simulink library "drr"  (Simulink 8.1)
settings: Solver=ode1  StartTime=0.0  StopTime=Inf  FixedStep=0.001  RelTol=1e-3
PostLoadFcn:
  | , if any(exist('dsrtsu_mdlpostloadfcn', 'file') == [2, 3, 6]), try dsrtsu_mdlpostloadfcn('Execute', bdroot); catch fprintf('Error in PostLoadFcn (dsrtsu_mdlpostloadfcn) for model "%s":\n %s\n', bdroot, lasterr); end, end,
undefined symbols (not defined in the file or in its folder): C_TICK_TIME_S, FALSE, KACC_ACCDecelIncLongTimer_s, KACC_ACCDecelIncMedTimer_s, KACC_ACCDecelIncShortTimer_s, KACC_ACCDecelIncSteps_num, KACC_ACCMCHardBrakingThrs_mps2, KACC_ACCMinSetTimeGap_s, KACC_BTSDecelRampDownRollAvgInt_s, KACC_DecelRampDownRollAvgInt_s, KACC_TargetDecelMargin_mps2, KACC_TimeGapIntrusionPerc_perc, TRUE, ZERO_FLOAT, ZERO_INT
libraries: hcu_lib x1, ltd x1
settings Model: DSRTSU_INTERNAL_RTI_VER=450  DSRTSU_INTERNAL_RTI_TYPE=rti1401  RTICANMMDATA=struct('GeneralSetupData',struct('modelroot','D:\ELN150201_TAIWAN\trunk\AdasDragon\software\sw_development\arch\app\acc','generalsettings',struct('filesettings',struct('destfolder',struct('Name','RTICANMM_FILES','Check',1),'buildfolder',struct('Name','.','Check',1),'AbsDestfolder',struct('Name','D:\ELN150201_TAIWAN\trunk\AdasDragon\software\sw_development\arch\app\acc\RTICANMM_FILES'),'AbsBuildfolder',struct('Name','D:\ELN150201_TAIWAN\trunk\AdasDragon\software\sw_development\arch\app\acc'))),'options',struct('addpaths',1,'rmpaths',1,'addtrcexclusion',logical(1),'cannavigator',struct('checkmonitoring',0),'show_usrtrc',0,'use_usrtrc',0),'advanced',struct('options',[1 1 1 1 1 1 1 1 1 1 1 1 1 1 1 1 1 1 1 1 1 1 1 1 1 1 1 1 1 1 1 1 1 1 1 1 1 1 1 1 1 1 1 1 1 1 1 1 1 1 1 1 1 1 1 1 1 1 1 1 1 1 1 1 1 1 1 1 1 1 1 1 1 1 1 1 1 1 1 1 1 1 1 1 1 1 1 1 1 1 1 1 1 1 1 1 1 1 1 1]),'MPSetup',{{}},'modelname','drr','block','drr'))  DSRTSU_INTERNAL_RTIFPGA=40  Creator=AT015411  LastModifiedBy=AT015555

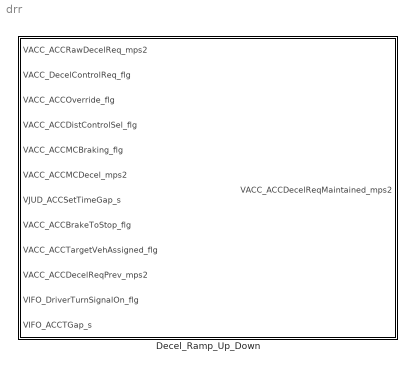
== system drr ==
  Decel_Ramp_Up_Down : Subsystem

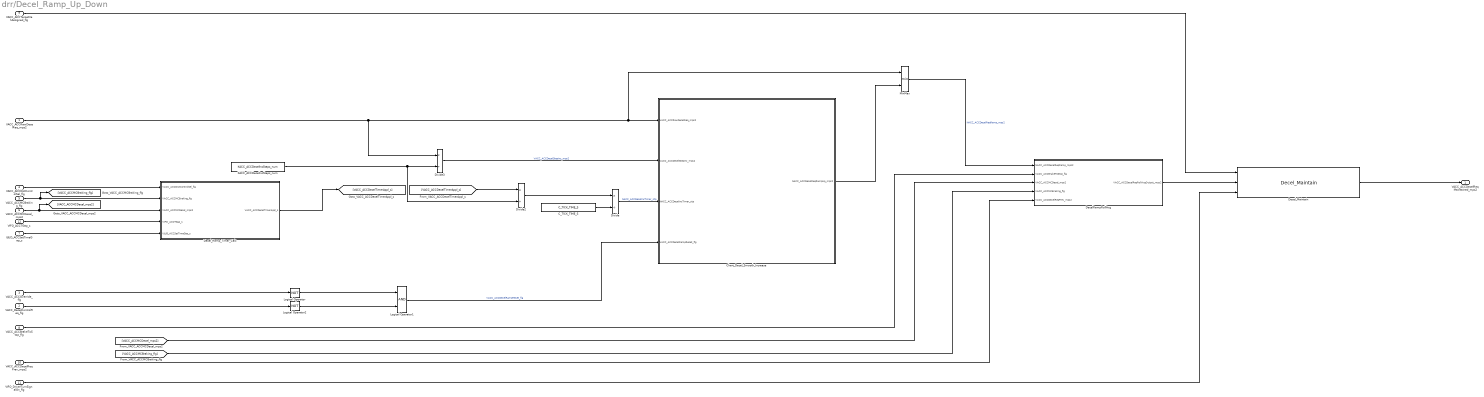
== system drr/Decel_Ramp_Up_Down ==
  VACC_ACCRawDecelReq_mps2 : Inport
  VACC_DecelControlReq_flg : Inport  Port=2
  VACC_ACCOverride_flg : Inport  Port=3
  VACC_ACCDistControlSel_flg : Inport  Port=4
  VACC_ACCMCBraking_flg : Inport  Port=5
  VACC_ACCMCDecel_mps2 : Inport  Port=6
  VJUD_ACCSetTimeGap_s : Inport  Port=7
  VACC_ACCBrakeToStop_flg : Inport  Port=8
  VACC_ACCTargetVehAssigned_flg : Inport  Port=9
  VACC_ACCDecelReqPrev_mps2 : Inport  Port=10
  VIFO_DriverTurnSignalOn_flg : Inport  Port=11
  VIFO_ACCTGap_s : Inport  Port=12
  C_TICK_TIME_S : Constant  Value=C_TICK_TIME_S
  Chart_Decel_Smooth_Increase : Stateflow chart  TreatAsAtomicUnit=on
  DecelRampRollAvg : Subsystem
  Decel_Maintain : ltd/Decel_Maintain
  Decel_Ramp_Timer_Calc : Subsystem
  Divide : Product  Inputs=*/
  Divide2 : Product  Inputs=*/
  Divide3 : Product  Inputs=*/
  KACC_ACCDecelIncSteps_num : Constant  Value=KACC_ACCDecelIncSteps_num
  Logical Operator : Logic  Operator=NOT  AllPortsSameDT=off  OutDataTypeStr=boolean
  Logical Operator1 : Logic  AllPortsSameDT=off  OutDataTypeStr=boolean
  Logical Operator2 : Logic  Operator=NOT  AllPortsSameDT=off  OutDataTypeStr=boolean
  MinMax : MinMax  Inputs=2
  VACC_ACCDecelReqMaintained_mps2 : Outport
  wires:
  Logical Operator2/1 -> Logical Operator1/2
  Chart_Decel_Smooth_Increase/1(NACC_ACCDecelReqRampUp_mps2) -> MinMax/2
  Divide3/1 -> Chart_Decel_Smooth_Increase/2(VACC_ACCDecelStepInc_mps2)  "VACC_ACCDecelStepInc_mps2"
  KACC_ACCDecelIncSteps_num/1 -> Divide2/2, Divide3/2
  Divide/1 -> Chart_Decel_Smooth_Increase/3(NACC_ACCDecelIncTimer_stp)  "NACC_ACCDecelIncTimer_stp"
  C_TICK_TIME_S/1 -> Divide/2
  Divide2/1 -> Divide/1
  VACC_ACCRawDecelReq_mps2/1 -> Divide3/1, MinMax/1, Chart_Decel_Smooth_Increase/1(VACC_ACCRawDecelReq_mps2)
  Logical Operator1/1 -> Chart_Decel_Smooth_Increase/4(VACC_ACCDecelRampReset_flg)  "VACC_ACCDecelRampReset_flg"
  VACC_ACCOverride_flg/1 -> Logical Operator/1
  Logical Operator/1 -> Logical Operator1/1
  VACC_DecelControlReq_flg/1 -> Logical Operator2/1
  [VACC_ACCDecelTimerAppl_s] -> Divide2/1
  VACC_ACCDistControlSel_flg/1 -> Decel_Ramp_Timer_Calc/1(VACC_ACCDistControlSel_flg)
  VIFO_ACCTGap_s/1 -> Decel_Ramp_Timer_Calc/4(VIFO_ACCTGap_s)
  VACC_ACCMCDecel_mps2/1 -> [VACC_ACCMCDecel_mps2], Decel_Ramp_Timer_Calc/3(VACC_ACCMCDecel_mps2)
  VJUD_ACCSetTimeGap_s/1 -> Decel_Ramp_Timer_Calc/5(VJUD_ACCSetTimeGap_s)
  VACC_ACCMCBraking_flg/1 -> [VACC_ACCMCBraking_flg], Decel_Ramp_Timer_Calc/2(VACC_ACCMCBraking_flg)
  Decel_Ramp_Timer_Calc/1(VACC_ACCDecelTimerAppl_s) -> [VACC_ACCDecelTimerAppl_s]
  VACC_ACCBrakeToStop_flg/1 -> DecelRampRollAvg/2(VACC_ACCBrakeToStop_flg)
  MinMax/1 -> DecelRampRollAvg/1(NACC_ACCDecelReqRamp_mps2)  "NACC_ACCDecelReqRamp_mps2"
  VACC_ACCTargetVehAssigned_flg/1 -> Decel_Maintain/1
  [VACC_ACCMCDecel_mps2] -> DecelRampRollAvg/3(VACC_ACCMCDecel_mps2)
  VACC_ACCDecelReqPrev_mps2/1 -> DecelRampRollAvg/5(VACC_ACCDecelReqPrev_mps2)
  DecelRampRollAvg/1(VACC_ACCDecelReqRollAvgOutput_mps2) -> Decel_Maintain/2
  Decel_Maintain/1 -> VACC_ACCDecelReqMaintained_mps2/1
  VIFO_DriverTurnSignalOn_flg/1 -> Decel_Maintain/3
  [VACC_ACCMCBraking_flg] -> DecelRampRollAvg/4(VACC_ACCMCBraking_flg)

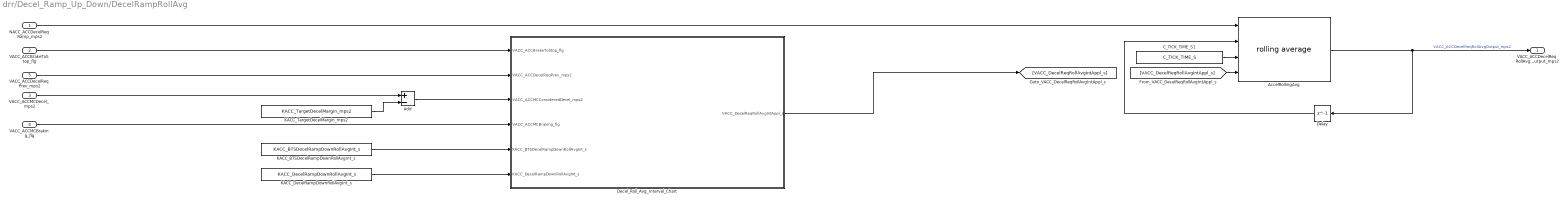
== system drr/Decel_Ramp_Up_Down/DecelRampRollAvg ==
  NACC_ACCDecelReqRamp_mps2 : Inport
  VACC_ACCBrakeToStop_flg : Inport  Port=2
  VACC_ACCMCDecel_mps2 : Inport  Port=3
  VACC_ACCMCBraking_flg : Inport  Port=4
  VACC_ACCDecelReqPrev_mps2 : Inport  Port=5
  AccelRollingAvg : hcu_lib/rolling average
  Add : Sum  Inputs=+-
  C_TICK_TIME_S1 : Constant  Value=C_TICK_TIME_S
  Decel_Roll_Avg_Interval_Chart : Stateflow chart  TreatAsAtomicUnit=on
  Delay : Delay  DelayLength=1
  KACC_BTSDecelRampDownRollAvgInt_s : Constant  Value=KACC_BTSDecelRampDownRollAvgInt_s
  KACC_DecelRampDownRollAvgInt_s : Constant  Value=KACC_DecelRampDownRollAvgInt_s
  KACC_TargetDecelMargin_mps2 : Constant  Value=KACC_TargetDecelMargin_mps2  OutDataTypeStr=single
  VACC_ACCDecelReqRollAvgOutput_mps2 : Outport
  wires:
  Delay/1 -> AccelRollingAvg/2
  KACC_DecelRampDownRollAvgInt_s/1 -> Decel_Roll_Avg_Interval_Chart/6(KACC_DecelRampDownRollAvgInt_s)
  C_TICK_TIME_S1/1 -> AccelRollingAvg/3
  NACC_ACCDecelReqRamp_mps2/1 -> AccelRollingAvg/1
  AccelRollingAvg/1 -> VACC_ACCDecelReqRollAvgOutput_mps2/1, Delay/1  "VACC_ACCDecelReqRollAvgOutput_mps2"
  VACC_ACCBrakeToStop_flg/1 -> Decel_Roll_Avg_Interval_Chart/1(VACC_ACCBrakeToStop_flg)
  KACC_BTSDecelRampDownRollAvgInt_s/1 -> Decel_Roll_Avg_Interval_Chart/5(KACC_BTSDecelRampDownRollAvgInt_s)
  [VACC_DecelReqRollAvgIntAppl_s] -> AccelRollingAvg/4
  VACC_ACCMCDecel_mps2/1 -> Add/1
  VACC_ACCDecelReqPrev_mps2/1 -> Decel_Roll_Avg_Interval_Chart/2(VACC_ACCDecelReqPrev_mps2)
  Decel_Roll_Avg_Interval_Chart/1(VACC_DecelReqRollAvgIntAppl_s) -> [VACC_DecelReqRollAvgIntAppl_s]
  KACC_TargetDecelMargin_mps2/1 -> Add/2
  Add/1 -> Decel_Roll_Avg_Interval_Chart/3(VACC_ACCMCConsideredDecel_mps2)
  VACC_ACCMCBraking_flg/1 -> Decel_Roll_Avg_Interval_Chart/4(VACC_ACCMCBraking_flg)

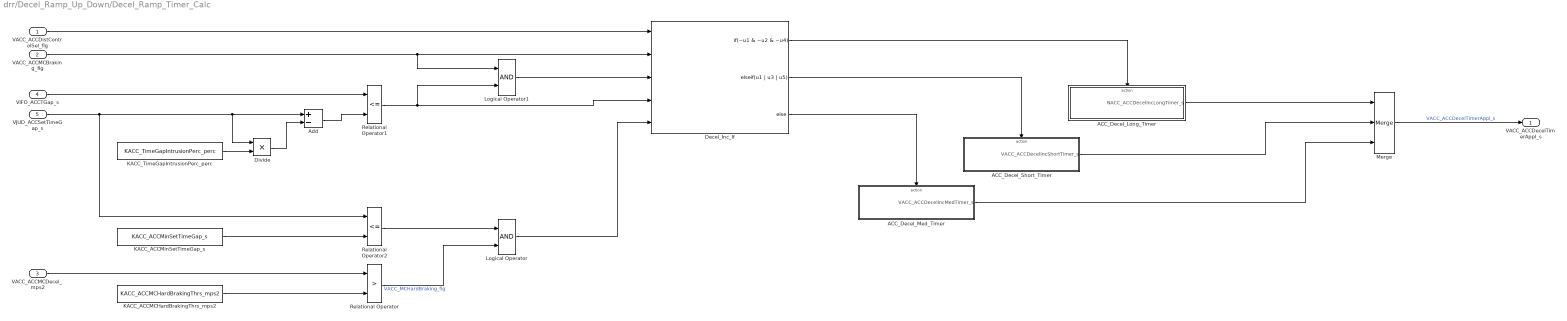
== system drr/Decel_Ramp_Up_Down/Decel_Ramp_Timer_Calc ==
  VACC_ACCDistControlSel_flg : Inport
  VACC_ACCMCBraking_flg : Inport  Port=2
  VACC_ACCMCDecel_mps2 : Inport  Port=3
  VIFO_ACCTGap_s : Inport  Port=4
  VJUD_ACCSetTimeGap_s : Inport  Port=5
  ACC_Decel_Long_Timer : Subsystem  TreatAsAtomicUnit=on
  ACC_Decel_Med_Timer : Subsystem  TreatAsAtomicUnit=on
  ACC_Decel_Short_Timer : Subsystem  TreatAsAtomicUnit=on
  Add : Sum  Inputs=+-
  Decel_Inc_If : If  NumInputs=5  IfExpression=~u1 & ~u2 & ~u4  ElseIfExpressions=u1 | u3 | u5
  Divide : Product  Inputs=**
  KACC_ACCMCHardBrakingThrs_mps2 : Constant  Value=KACC_ACCMCHardBrakingThrs_mps2
  KACC_ACCMinSetTimeGap_s : Constant  Value=KACC_ACCMinSetTimeGap_s
  KACC_TimeGapIntrusionPerc_perc : Constant  Value=KACC_TimeGapIntrusionPerc_perc
  Logical Operator : Logic  AllPortsSameDT=off  OutDataTypeStr=boolean
  Logical Operator1 : Logic  AllPortsSameDT=off  OutDataTypeStr=boolean
  Merge : Merge  Inputs=3
  Relational Operator : RelationalOperator  Operator=>  OutDataTypeStr=boolean
  Relational Operator1 : RelationalOperator  Operator=<=  OutDataTypeStr=boolean
  Relational Operator2 : RelationalOperator  Operator=<=  OutDataTypeStr=boolean
  VACC_ACCDecelTimerAppl_s : Outport
  wires:
  VACC_ACCMCDecel_mps2/1 -> Relational Operator/1
  KACC_ACCMCHardBrakingThrs_mps2/1 -> Relational Operator/2
  VIFO_ACCTGap_s/1 -> Relational Operator1/1
  VJUD_ACCSetTimeGap_s/1 -> Add/1, Divide/1, Relational Operator2/1
  KACC_ACCMinSetTimeGap_s/1 -> Relational Operator2/2
  VACC_ACCDistControlSel_flg/1 -> Decel_Inc_If/1
  VACC_ACCMCBraking_flg/1 -> Logical Operator1/1, Decel_Inc_If/2
  Relational Operator/1 -> Logical Operator/2  "VACC_MCHardBraking_flg"
  Relational Operator1/1 -> Decel_Inc_If/4, Logical Operator1/2
  Relational Operator2/1 -> Logical Operator/1
  Decel_Inc_If/1 -> ACC_Decel_Long_Timer/Action
  Logical Operator/1 -> Decel_Inc_If/5
  Decel_Inc_If/2 -> ACC_Decel_Short_Timer/Action
  Decel_Inc_If/3 -> ACC_Decel_Med_Timer/Action
  Merge/1 -> VACC_ACCDecelTimerAppl_s/1  "VACC_ACCDecelTimerAppl_s"
  ACC_Decel_Long_Timer/1(NACC_ACCDecelIncLongTimer_s) -> Merge/1
  ACC_Decel_Short_Timer/1(VACC_ACCDecelIncShortTimer_s) -> Merge/2
  ACC_Decel_Med_Timer/1(VACC_ACCDecelIncMedTimer_s) -> Merge/3
  Logical Operator1/1 -> Decel_Inc_If/3
  KACC_TimeGapIntrusionPerc_perc/1 -> Divide/2
  Add/1 -> Relational Operator1/2
  Divide/1 -> Add/2

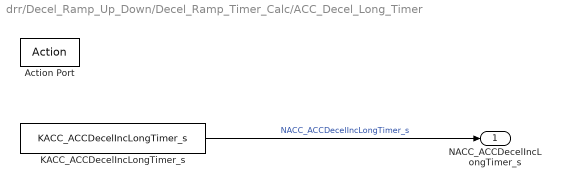
== system drr/Decel_Ramp_Up_Down/Decel_Ramp_Timer_Calc/ACC_Decel_Long_Timer ==
  Action Port : ActionPort  ActionType=then
  KACC_ACCDecelIncLongTimer_s : Constant  Value=KACC_ACCDecelIncLongTimer_s
  NACC_ACCDecelIncLongTimer_s : Outport
  wires:
  KACC_ACCDecelIncLongTimer_s/1 -> NACC_ACCDecelIncLongTimer_s/1  "NACC_ACCDecelIncLongTimer_s"

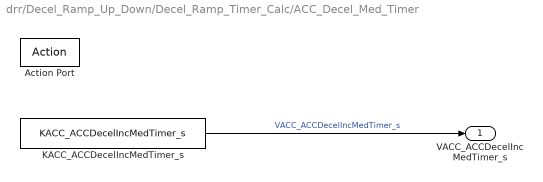
== system drr/Decel_Ramp_Up_Down/Decel_Ramp_Timer_Calc/ACC_Decel_Med_Timer ==
  Action Port : ActionPort  ActionType=else
  KACC_ACCDecelIncMedTimer_s : Constant  Value=KACC_ACCDecelIncMedTimer_s
  VACC_ACCDecelIncMedTimer_s : Outport
  wires:
  KACC_ACCDecelIncMedTimer_s/1 -> VACC_ACCDecelIncMedTimer_s/1  "VACC_ACCDecelIncMedTimer_s"

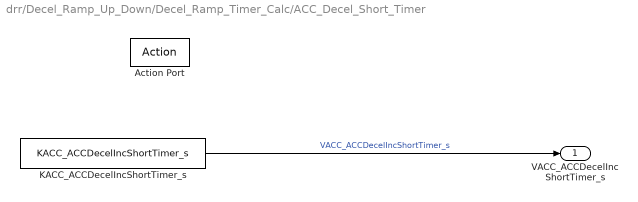
== system drr/Decel_Ramp_Up_Down/Decel_Ramp_Timer_Calc/ACC_Decel_Short_Timer ==
  Action Port : ActionPort  ActionType=elseif
  KACC_ACCDecelIncShortTimer_s : Constant  Value=KACC_ACCDecelIncShortTimer_s
  VACC_ACCDecelIncShortTimer_s : Outport
  wires:
  KACC_ACCDecelIncShortTimer_s/1 -> VACC_ACCDecelIncShortTimer_s/1  "VACC_ACCDecelIncShortTimer_s"

== stateflow chart Decel_Ramp_Up_Down/DecelRampRollAvg/Decel_Roll_Avg_Interval_Chart ==
  state DECEL_SHORT_INTERVAL
    en:
    VACC_DecelReqRollAvgIntAppl_s=KACC_DecelRampDownRollAvgInt_s;
  state DECEL_LONG_INTERVAL
    en:
    VACC_DecelReqRollAvgIntAppl_s=KACC_BTSDecelRampDownRollAvgInt_s;
  (default) -> DECEL_SHORT_INTERVAL
  DECEL_SHORT_INTERVAL -> DECEL_LONG_INTERVAL : [VACC_ACCBrakeToStop_flg==TRUE...
      | && VACC_ACCDecelReqPrev_mps2 > VACC_ACCMCConsideredDecel_mps2...
      | && VACC_ACCMCBraking_flg==TRUE]
  DECEL_LONG_INTERVAL -> DECEL_SHORT_INTERVAL : [VACC_ACCBrakeToStop_flg==FALSE]
  data: VACC_DecelReqRollAvgIntAppl_s output single; VACC_ACCBrakeToStop_flg input double; VACC_ACCDecelReqPrev_mps2 input double; VACC_ACCMCConsideredDecel_mps2 input double; VACC_ACCMCBraking_flg input double; KACC_BTSDecelRampDownRollAvgInt_s input double; KACC_DecelRampDownRollAvgInt_s input double; TRUE parameter boolean; FALSE parameter boolean

== stateflow chart Decel_Ramp_Up_Down/Chart_Decel_Smooth_Increase ==
  state INIT
    en:
    NACC_ACCDecelReqRampUp_mps2 = ZERO_FLOAT;
  state COUNT
    en:
    NACC_ACCDecelIncTimerLocal_stp=ZERO_INT;
    du:
    NACC_ACCDecelIncTimerLocal_stp=NACC_ACCDecelIncTimerLocal_stp+1;
  state INC_DECEL
    en:
    NACC_ACCDecelReqRampUp_mps2=NACC_ACCDecelReqRampUp_mps2+VACC_ACCDecelStepInc_mps2;
  (default) -> INIT
  COUNT -> INC_DECEL [order 1] : [NACC_ACCDecelIncTimerLocal_stp>NACC_ACCDecelIncTimer_stp]
  INIT -> COUNT : [NACC_ACCDecelReqRampUp_mps2<VACC_ACCRawDecelReq_mps2]
  INC_DECEL -> COUNT [order 1] : [NACC_ACCDecelReqRampUp_mps2<VACC_ACCRawDecelReq_mps2]
  COUNT -> INIT [order 2] : [VACC_ACCDecelRampReset_flg==TRUE]
  INC_DECEL -> INIT [order 2] : [VACC_ACCDecelRampReset_flg==TRUE]
  data: VACC_ACCRawDecelReq_mps2 input double; VACC_ACCDecelStepInc_mps2 input double; NACC_ACCDecelIncTimer_stp input double; NACC_ACCDecelReqRampUp_mps2 output single; ZERO_FLOAT parameter single; NACC_ACCDecelIncTimerLocal_stp local single; ZERO_INT parameter uint8; VACC_ACCDecelRampReset_flg input double; TRUE parameter boolean
